simulink model "Fig44"  (R2014b)
settings: Solver=FixedStepDiscrete  StartTime=0.0  StopTime=.005  RelTol=1e-3
libraries: dspsigops x1
settings Model: Creator=Dennis Silage  LastModifiedBy=Silage
settings DataIOCC: SignalLoggingSaveFormat=ModelDataLogs
settings OptimizationCC: ExpressionDepthLimit=2147483647  InitFltsAndDblsToZero=on
settings DebuggingCC: UnderspecifiedInitializationDetection=Classic  MergeDetectMultiDrivingBlocksExec=none  FcnCallInpInsideContextMsg=UseLocalSettings  StateNameClashWarn=warning  StrictBusMsg=Warning
settings GRTTargetCC: CombineOutputUpdateFcns=off  GRTInterface=on

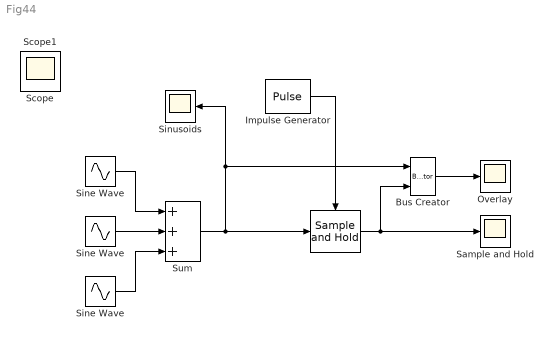
== system Fig44 ==
  "   " : dspsigops/Sample and Hold  trig=Rising edge  initCond=0  latchinput=off
  " Sine Wave " : Sin  Amplitude=0.2  Frequency=5000*pi  SampleTime=1.25e-6
  Bus Creator : BusCreator  Inputs=2
  Impulse Generator : DiscretePulseGenerator  Period=100  SampleTime=1.25e-6
  Overlay : Scope
      settings: YMin=-1.5  YMax=1.5  SaveName=ScopeData5
  "Sample and Hold " : Scope
      settings: YMin=-1.5  YMax=1.5  SaveName=ScopeData3
  Sine Wave : Sin  Frequency=1000*pi  SampleTime=1.25e-6
  "Sine Wave " : Sin  Amplitude=0.5  Frequency=3000*pi  SampleTime=1.25e-6
  Sinusoids : Scope
      settings: YMin=-1.5  YMax=1.5
  Sum : Sum  Inputs=+++
  Scope : Scope
      settings: MaxDataPoints=7500  SampleTime=-1
  Scope1 : Scope
      settings: MaxDataPoints=7500  SampleTime=-1
  wires:
  "Sine Wave "/1 -> Sum/2
  " Sine Wave "/1 -> Sum/3
  Sine Wave/1 -> Sum/1
  Sum/1 -> "   "/1, Sinusoids/1, Bus Creator/1
  Impulse Generator/1 -> "   "/Trigger
  "   "/1 -> "Sample and Hold "/1, Bus Creator/2
  Bus Creator/1 -> Overlay/1
